simulink model "Check_alpha_beta_from_quaternions"  (R2016a)
settings: Solver=ode4  StartTime=0.0  StopTime=10.0  FixedStep=0.001  RelTol=1e-3
libraries: aerolibconvert2 x3, aerolibtransform2 x1
settings Model: Creator=PD Banneheka  LastModifiedBy=PD Banneheka
settings GRTTargetCC: GeneratePreprocessorConditionals=Use local settings

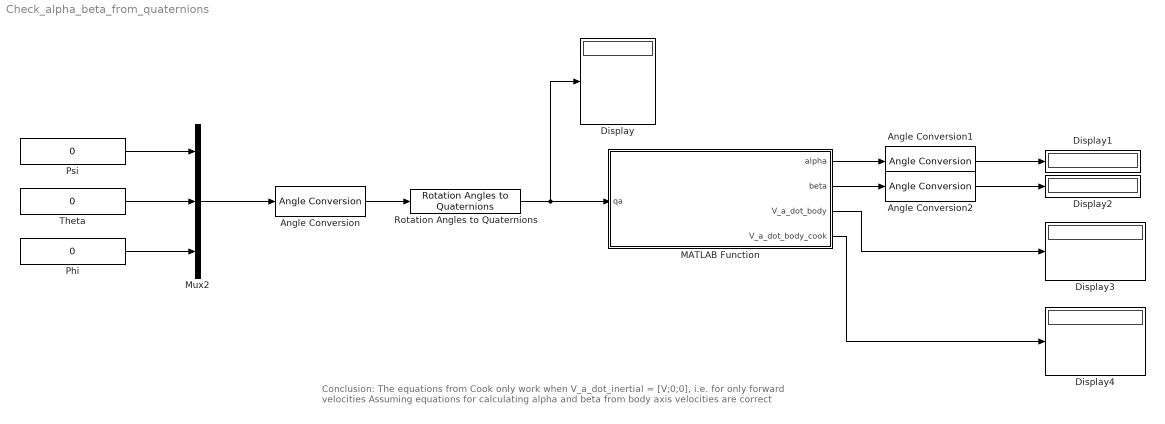
== system Check_alpha_beta_from_quaternions ==
  note: Conclusion:
      |
      | The equations from Cook only work when V_a_dot_inertial = [V;0;0], i.e. for only forward velocities
      |
      | Assuming equations for calculating alpha and beta from body axis velocities are correct
  Angle Conversion : aerolibconvert2/Angle Conversion  IU=deg  OU=rad
  Angle Conversion1 : aerolibconvert2/Angle Conversion  IU=rad  OU=deg
  Angle Conversion2 : aerolibconvert2/Angle Conversion  IU=rad  OU=deg
  Display{,1..4} (5 alike) : Display
  MATLAB Function : MATLAB Function  TreatAsAtomicUnit=on
  Mux2 : Mux  Inputs=3
  Phi : Constant  Value=0
  Psi : Constant  Value=0
  Rotation Angles to Quaternions : aerolibtransform2/Rotation Angles to Quaternions  rotationOrder=ZYX
  Theta : Constant  Value=0
  wires:
  Psi/1 -> Mux2/1
  Rotation Angles to Quaternions/1 -> MATLAB Function/1(qa), Display/1
  Angle Conversion/1 -> Rotation Angles to Quaternions/1
  Theta/1 -> Mux2/2
  Mux2/1 -> Angle Conversion/1
  Phi/1 -> Mux2/3
  MATLAB Function/1(alpha) -> Angle Conversion1/1
  MATLAB Function/2(beta) -> Angle Conversion2/1
  Angle Conversion1/1 -> Display1/1
  Angle Conversion2/1 -> Display2/1
  MATLAB Function/3(V_a_dot_body) -> Display3/1
  MATLAB Function/4(V_a_dot_body_cook) -> Display4/1

== matlab function Check_alpha_beta_from_quaternions/MATLAB Function ==
  data: qa input; alpha output; beta output; V_a_dot_body output; V_a_dot_body_cook output
function [alpha,beta,V_a_dot_body,V_a_dot_body_cook]= fcn(qa)
% Velocity of aircraft in inertial axes
qa_dot = [  0
            0
            10  ];

V_t = 30; % Tunnel windspeed (m/s)

%% Transformation matrices

% Quaternion parameters (for phi=10deg, theta=20deg, psi=30deg, 
% found using "Rotation Angles to Quaternions" block with rotation order ZYX
% where first angle input is psi, second is theta, and third is phi,
% i.e. aircraft attitude rotation squence from inertial axis to body axis is yaw, pitch, roll)
% qa0 = 0.9515;
% qa1 = 0.03813;
% qa2 = 0.1893;
% qa3 = 0.2393;

% Taking values of quaternion parameters directly from block
qa0 = qa(1);
qa1 = qa(2);
qa2 = qa(3);
qa3 = qa(4);

Ea = [  -qa1     qa0      -qa3     qa2
        -qa2     qa3      qa0      -qa1
        -qa3     -qa2     qa1      qa0  ];
    
E_dasha = [     -qa1     qa0      qa3      -qa2
                -qa2     -qa3     qa0      qa1
                -qa3     qa2      -qa1     qa0  ];
            
Aa = Ea*transpose(E_dasha);

%% Calculating angle of attack (alpha), sideslip (sideslip) and local angular velocities (p, q, r)

% Velocity of aircraft in inertial axes
V_a_dot_inertial = [    qa_dot(1)+V_t
                        qa_dot(2)
                        qa_dot(3)      ];

% Velocity of aircraft in body axes (vector_inertial = A * vector_body, where A is the transformation matrix)
V_a_dot_body = transpose(Aa)*V_a_dot_inertial;

% Magnitude of total local velocity vector
V = sqrt((V_a_dot_inertial(1))^2+(V_a_dot_inertial(2))^2+(V_a_dot_inertial(3))^2);

% Angle of attack (alpha)
alpha = atan2(V_a_dot_body(3),V_a_dot_body(1));

% Sideslip angle (beta)
beta = asin(V_a_dot_body(2)/V);

%% Comparing V_a_dot_body with that obtained from transformation in Cook (page 22)
V_a_dot_body_cook = [   cos(alpha)*cos(beta)    -cos(alpha)*sin(beta)   -sin(alpha)
                        sin(beta)               cos(beta)               0
                        sin(alpha)*cos(beta)    -sin(alpha)*sin(beta)   cos(alpha)  ]   *   [V_a_dot_inertial];
